simulink model "QuadrotorModel"  (R2023b)
settings: Solver=VariableStepAuto  StartTime=0.0  StopTime=100  RelTol=1e-3
settings Model: Creator=hp  LastModifiedBy=hp

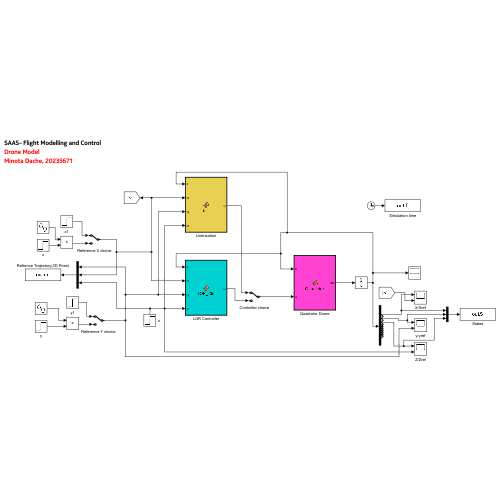
[thumbnail: Simulink's stored preview of the top-level diagram]
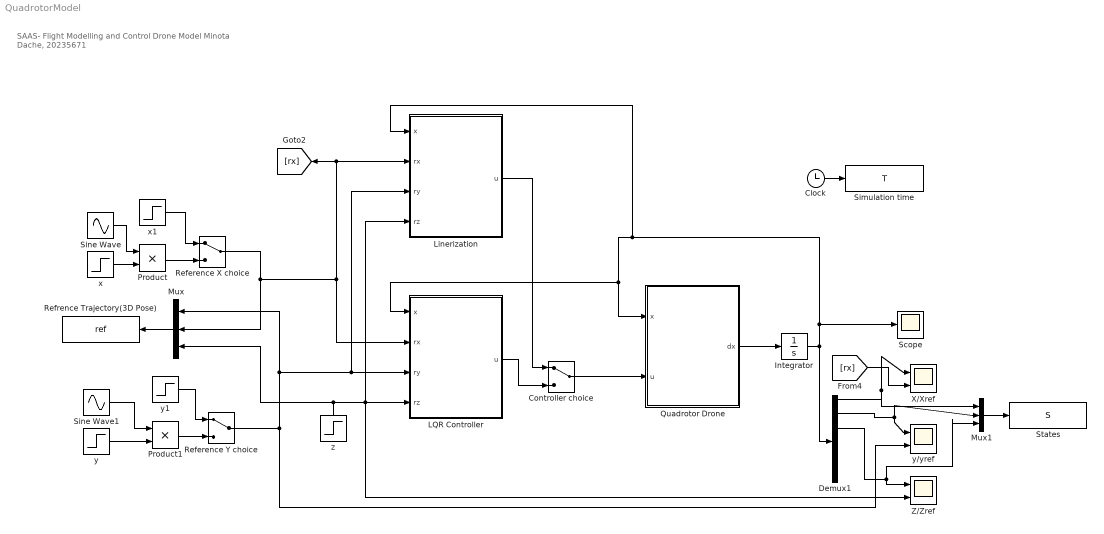
== system QuadrotorModel ==
  note: SAAS- Flight Modelling and Control
      | Drone Model
      | Minota Dache, 20235671
  Clock : Clock
  Controller choice : ManualSwitch
  Demux1 : Demux  Outputs=12
  Integrator : Integrator
  LQR Controller : MATLAB Function  TreatAsAtomicUnit=on
  Linerization : MATLAB Function  TreatAsAtomicUnit=on
  Mux : Mux  Inputs=3
  Mux1 : Mux  Inputs=3
  Product : Product
  Product1 : Product
  Quadrotor Drone : MATLAB Function  TreatAsAtomicUnit=on
  Reference X choice : ManualSwitch
  Reference Y choice : ManualSwitch
  Refrence Trajectory(3D Pose) : ToWorkspace  VariableName=ref  SampleTime=-1
  Scope : Scope
  Simulation time : ToWorkspace  VariableName=T  SampleTime=-1
  Sine Wave : Sin  Frequency=0.05  SampleTime=0
  Sine Wave1 : Sin  Frequency=0.05  SampleTime=0
  States : ToWorkspace  VariableName=S  SampleTime=-1
  X/Xref : Scope  NumInputPorts=2
  Z/Zref : Scope  NumInputPorts=2
  x : Step  Time=10  SampleTime=0
  x1 : Step  Time=10  SampleTime=0
  y : Step  Time=20  SampleTime=0
  y/yref : Scope  NumInputPorts=2
  y1 : Step  Time=10  SampleTime=0
  z : Step  SampleTime=0
  wires:
  Linerization/1(u) -> Controller choice/1
  LQR Controller/1(u) -> Controller choice/2
  Controller choice/1 -> Quadrotor Drone/2(u)
  Quadrotor Drone/1(dx) -> Integrator/1
  Sine Wave/1 -> Product/1
  x/1 -> Product/2
  y/1 -> Product1/2
  Sine Wave1/1 -> Product1/1
  x1/1 -> Reference X choice/1
  Product/1 -> Reference X choice/2
  Product1/1 -> Reference Y choice/2
  y1/1 -> Reference Y choice/1
  Mux/1 -> Refrence Trajectory(3D Pose)/1
  Reference X choice/1 -> Mux/2, Linerization/2(rx), [rx], LQR Controller/2(rx)
  Integrator/1 -> Demux1/1, Scope/1, Linerization/1(x), LQR Controller/1(x), Quadrotor Drone/1(x)
  Clock/1 -> Simulation time/1
  z/1 -> Mux/3, Z/Zref/2, LQR Controller/4(rz), Linerization/4(rz)
  Reference Y choice/1 -> Mux/1, LQR Controller/3(ry), Linerization/3(ry), y/yref/2
  [rx] -> X/Xref/2
  Mux1/1 -> States/1
  Demux1/1 -> Mux1/1, X/Xref/1
  Demux1/3 -> Mux1/2, y/yref/1
  Demux1/5 -> Mux1/3, Z/Zref/1

== matlab function QuadrotorModel/LQR Controller ==
  data: x input; rx input; u output; ry input; rz input
function u = LQR_Ctrl(x,rx,ry,rz)
%#codegen

u = zeros(6,1);

g  = 9.81;

% les moments inirtiels 
Ixx=7.5*10^-3;
Iyy=7.5*10^-3;
Izz=1.3*10^-3;

k1 = 2; k2 = 3;
k3 = 3; k4 = 5;
k5 = 2; k6 = 4;
k7 = 2; k8 = 3;
k9 = 2; k10 = 6;
k11 = 2; k12 = 3;

% les coeficients 
a1=((Iyy-Izz)/Ixx);
a2=((Izz-Ixx)/Iyy);
a3=((Ixx-Iyy)/Izz);

Lqr_x = [-1.0000   -2.0815   16.3461    7.7992];
Lqr_y = [1.0000    1.7953   10.9036    3.2848];



u(1) = -Lqr_x*[x(1)-rx;x(2);x(9);x(10)] ;
u(2) = -Lqr_y*[x(3)-ry;x(4);x(7);x(8)];
u(3) = -(x(10)*x(2)-x(8)*x(4)+g*cos(x(7))*cos(x(9)))-k5*(x(5)-rz)-k6*x(6);
u(4) = -(a1*x(12)*x(10))-k7*x(7)-k8*x(8);
u(5) = -a2*x(12)*x(8)-k9*x(9)-k10*x(10);

== matlab function QuadrotorModel/Quadrotor Drone ==
  data: x input; u input; dx output
function dx = Quadrotor(x,u)
%#codegen

g  = 9.81;

% les moments inirtiels 
Ixx=7.5*10^-3;
Iyy=7.5*10^-3;
Izz=1.3*10^-3;


% les coeficients 
a1=((Iyy-Izz)/Ixx);
a2=((Izz-Ixx)/Iyy);
a3=((Ixx-Iyy)/Izz);

dx = zeros(12,1);

dx(1) = x(2);
dx(2) = x(12)*x(4)-x(10)*x(6)-g*sin(x(9))+u(1);
dx(3) = x(4);
dx(4) = x(8)*x(6)-x(12)*x(2)+g*sin(x(7))*cos(x(9))+u(2);
dx(5) = x(6);
dx(6) = x(10)*x(2)-x(8)*x(4)+g*cos(x(7))*cos(x(9))+u(3);
dx(7) = x(8);
dx(8) = a1*x(12)*x(10)+u(2);
dx(9) = x(10);
dx(10) = a2*x(12)*x(8)+u(1);
dx(11) = x(12);
dx(12) = a3*x(8)*x(10)+u(4)+u(5);

== matlab function QuadrotorModel/Linerization ==
  data: x input; rx input; u output; ry input; rz input
function u = fcn(x,rx,ry,rz)
%#codegen


u = zeros(6,1);

g  = 9.81;

% les moments inirtiels 
Ixx=7.5*10^-3;
Iyy=7.5*10^-3;
Izz=1.3*10^-3;

k1 = 2; k2 = 3;
k3 = 3; k4 = 5;
k5 = 2; k6 = 4;
k7 = 2; k8 = 3;
k9 = 2; k10 = 6;
k11 = 2; k12 = 3;

% les coeficients 
a1=((Iyy-Izz)/Ixx);
a2=((Izz-Ixx)/Iyy);
a3=((Ixx-Iyy)/Izz);

% ld1 = 2;
% ld2 = 2;
% s1=(x(2)-drx)+ld1*(x(1)-rx);
% s2=(x(4)-drx)+ld2*(x(3)-ry);

% u(1) = -(x(12)*x(4)-x(10)*x(6)-g*sin(x(9)))-ld1*(x(2)-drx)-k2*tanh(s1)+d2rx;
% u(2) = -(x(8)*x(6)-x(12)*x(2)+g*sin(x(7))*cos(x(9)))-ld2*(x(4)-dry)-k4*tanh(s2)+d2ry;
u(1) = -(x(12)*x(4)-x(10)*x(6)-g*sin(x(9)))-k1*(x(1)-rx)-k2*(x(2));
u(2) = -(x(8)*x(6)-x(12)*x(2)+g*sin(x(7))*cos(x(9)))-k3*(x(3)-ry)-k4*x(4);
u(3) = -(x(10)*x(2)-x(8)*x(4)+g*cos(x(7))*cos(x(9)))-k5*(x(5)-rz)-k6*x(6);
u(4) = -(a1*x(12)*x(10))-k7*x(7)-k8*x(8);
u(5) = -a2*x(12)*x(8)-k9*x(9)-k10*x(10);
